simulink model "EJ1_LazoCerradoSISO"  (R2018b)
settings: Solver=VariableStepAuto  StartTime=0.0  StopTime=2000  RelTol=1e-3  EnableMultiTasking=on
StartFcn:
  | clear all
undefined symbols (not defined in the file or in its folder): sigbuilder_block
libraries: realtime_pacer_lib x1
settings Model: Creator=johnh  LastModifiedBy=jarico
settings OptimizationCC: LifeSpan=inf
settings DebuggingCC: SFUnexpectedBacktrackingDiag=warning  SFNoUnconditionalDefaultTransitionDiag=warning  SFExecutionAtInitializationDiag=none
settings SFSimCC: SimUseLocalCustomCode=off
settings RTWCC: RTWUseLocalCustomCode=off
settings CodeAppCC: StateflowObjectComments=on
settings GRTTargetCC: TargetLangStandard=C89/C90 (ANSI)  GeneratePreprocessorConditionals=Disable all
settings ConfigComp: CovMetricSettings=dw  CovHtmlReporting=on  CovSaveCumulativeToWorkspaceVar=on  CovSaveSingleToWorkspaceVar=on  CovExternalEMLEnable=off

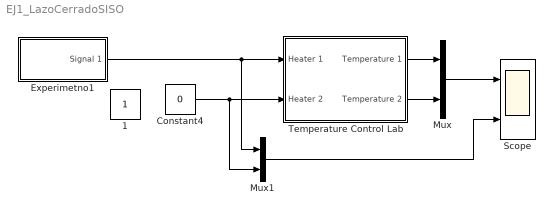
== system EJ1_LazoCerradoSISO ==
  Constant4 : Constant  Value=0
  Experimetno1 : Subsystem  Tag=STV Subsys  LoadFcn=sigbuilder_block('load');  StartFcn=sigbuilder_block('start');  StopFcn=sigbuilder_block('stop');  ClipboardFcn=sigbuilder_block('clipboard');  mask(Sigbuilder block){tuvar=[0:10]}
      mask help: Simulink:masks:SigbuilderBlock_MD
      mask init:
      | if ~strcmp(get_param(bdroot(gcbh),'SimulationStatus'),'stopped') tuvar = sigbuilder_block('maskInit'); end
      settings: CopyFcn=sigbuilder_block('copy');  DeleteFcn=sigbuilder_block('delete');  ModelCloseFcn=sigbuilder_block('modelClose');  PreSaveFcn=sigbuilder_block('preSave');  PauseFcn=sigbuilder_block('pause');  ContinueFcn=sigbuilder_block('continue');  NameChangeFcn=sigbuilder_block('namechange');  OpenFcn=sigbuilder_block('open',[408.75 447 551.25 400.5 ]);  CloseFcn=sigbuilder_block('close');
      mask Display: plot(0, 0, 100, 100,[2, 2, 32, 32, 2], [68, 8, 8, 68, 68],[32, 2], [38, 38], [32, 19, 2],[53, 60, 44], [32, 17, 17, 2],[16, 16, 31, 31]);txt = getActiveGroup(gcbh);text(2, 100, txt,'verticalAlignment', 'top');
  Mux : Mux  Inputs=2
  Mux1 : Mux  Inputs=2
  Scope : Scope  NumInputPorts=2
  Temperature Control Lab : Subsystem  mask(SISTEMA DE CONTROL DE TEMPERATURA){maxQ1=100, maxQ2=100, maxT1=60, maxT2=80, uLED=40}
      mask prompts: maxQ1 "Potencia máxima Q1 (%)"; maxQ2 "Potencia máxima Q2 (%)"; maxT1 "Temperatura máxima T1 (ºC)"; maxT2 "Temperatura máxima T2 (ºC)"; uLED "Temperatura umpral para indicadores luminosos (ºC)"
      mask help:
      | Ajuste la configuración del dispositivo en función de sus necesidades.
      | Por seguridad, se recomienda limitar la temperatura en los transistores a un valor máximo de 80ºC.
  1 : Constant  IOType=siggen
  wires:
  Temperature Control Lab/1(Temperature 1) -> Mux/1
  Constant4/1 -> Mux1/2, Temperature Control Lab/2(Heater 2)
  Temperature Control Lab/2(Temperature 2) -> Mux/2
  Mux/1 -> Scope/1
  Mux1/1 -> Scope/2
  Experimetno1/1(Signal 1) -> Mux1/1, Temperature Control Lab/1(Heater 1)

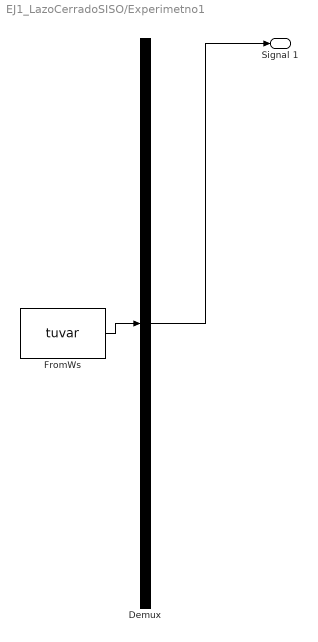
== system EJ1_LazoCerradoSISO/Experimetno1 ==
  Demux : Demux  Tag=STV Demux  Outputs=1
  FromWs : FromWorkspace  Tag=STV FromWs  VariableName=tuvar  SampleTime=0
      SigBuilderData=|
      | common.afterFinalStr = 'Extrapolate'
      | common.sampleTime = 0
      | dataSet.timeRange = [0 6100]
      | dataSet.name = 'Group 1'
      | sbobj.Groups.Name = 'Group 1'
      | sbobj.Groups.Signals.Name = 'Signal 1'
      | sbobj.Groups.Signals.XData = [0 50 50 1100 1100 2100 2100 3100 3100 4100 4100 5100 5100 6100]
      | sbobj.Groups.Signals.YData = [0 0 40 40 60 60 70 70 30 30 80 80 0 0]
      | sbobj.Groups.TimeRange = [0 6100]
  Signal 1 : Outport  Tag=STV Outport
  wires:
  FromWs/1 -> Demux/1
  Demux/1 -> Signal 1/1

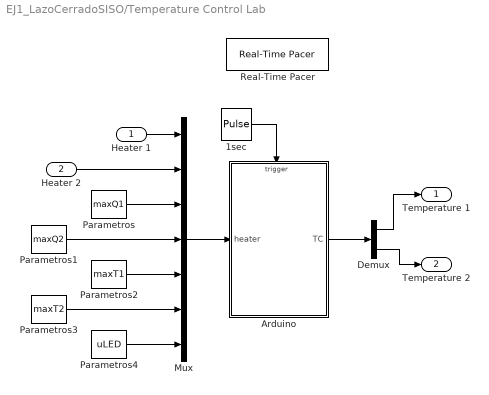
== system EJ1_LazoCerradoSISO/Temperature Control Lab ==
  Heater 1 : Inport
  Heater 2 : Inport  Port=2
  1sec : DiscretePulseGenerator  PulseType=Time based  Period=1  PulseWidth=50
  Arduino : Subsystem  TreatAsAtomicUnit=on
  Demux : Demux  Outputs=2
  Mux : Mux  Inputs=7
  Parametros : Constant  Value=maxQ1
  Parametros1 : Constant  Value=maxQ2
  Parametros2 : Constant  Value=maxT1
  Parametros3 : Constant  Value=maxT2
  Parametros4 : Constant  Value=uLED
  Real-Time Pacer : realtime_pacer_lib/Real-Time Pacer  simTimePerRealTime=1
  Temperature 1 : Outport
  Temperature 2 : Outport  Port=2
  wires:
  1sec/1 -> Arduino/Trigger
  Arduino/1(TC) -> Demux/1
  Heater 1/1 -> Mux/1
  Heater 2/1 -> Mux/2
  Mux/1 -> Arduino/1(heater)
  Demux/1 -> Temperature 1/1
  Demux/2 -> Temperature 2/1
  Parametros4/1 -> Mux/7
  Parametros3/1 -> Mux/6
  Parametros2/1 -> Mux/5
  Parametros1/1 -> Mux/4
  Parametros/1 -> Mux/3

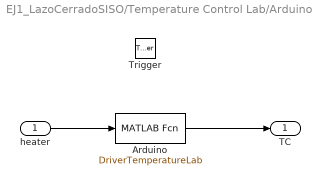
== system EJ1_LazoCerradoSISO/Temperature Control Lab/Arduino ==
  heater : Inport  LatchByDelayingOutsideSignal=on
  Trigger : TriggerPort  VariantControl=Variant
  Arduino : MATLABFcn  MATLABFcn=DriverTemperatureLab  OutputDimensions=2
  TC : Outport  InitialOutput=23
  wires:
  heater/1 -> Arduino/1
  Arduino/1 -> TC/1
